simulink model "rtwdemo_ValidateLegacyCodeVrsSim"  (Simulink 7.6)
settings: Solver=FixedStepDiscrete  StartTime=0.0  StopTime=4  FixedStep=.001  RelTol=1e-3
PostLoadFcn:
  | % Load data for this model
  | rtwdemo_legacyValidationData;
undefined symbols (not defined in the file or in its folder): P_InErrMap, P_OutMap
settings Model: Creator=The MathWorks Inc.  ExtModeAutoUpdateStatusClock=off
settings OptimizationCC: InitFltsAndDblsToZero=on
settings DebuggingCC: SignalResolutionControl=TryResolveAllWithWarning  StrictBusMsg=Warning
settings GRTTargetCC: TargetFcnLib=ansi_tfl_tmw.mat

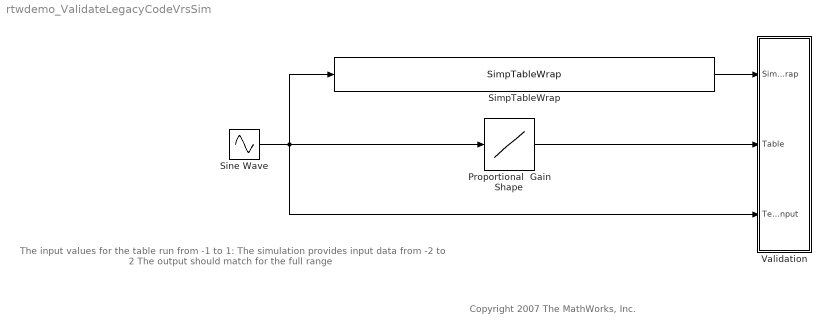
== system rtwdemo_ValidateLegacyCodeVrsSim ==
  note: The input values for the table run from -1 to 1:
      | The simulation provides input data from -2 to 2
      | The output should match for the full range
  note: Copyright 2007 The MathWorks, Inc.
  Proportional  Gain Shape : Lookup  InputValues=P_InErrMap  Table=P_OutMap  LookUpMeth=Interpolation-Use End Values
  SimpTableWrap : S-Function  FunctionName=SimpTableWrap  Parameters=SParameter1, SParameter2, SParameter3  EnableBusSupport=off  mask(Legacy Function){SFunctionSpec=double y1 = SimpleTable(double u1, double p1[], double p2[], int16 p3), SParameter1=P_InErrMap, SParameter2=P_OutMap, SParameter3=int16(length(P_OutMap)), ShowSpec=on}
      mask prompts: SParameter1 "P1:"; SParameter2 "P2:"; SParameter3 "P3:"; ShowSpec "Display function specification"
      mask help:
      | This block allows the user to call the following C function(s) in Simulink:
      |
      | StartFcn: none
      |
      | OutputFcn: double y1 = SimpleTable(double u1, double p1[], double p2[], int16 p3)
      |
      | TerminateFcn: none
      mask CallbackString:
      | ||||if strcmp(get_param(gcbh, 'ShowSpec'), 'on')
      |   set_param(gcbh, 'MaskDisplay', sprintf('fprintf(''%s'');', get_param(gcbh, 'SFunctionSpec')));
      | else
      |   set_param(gcbh, 'MaskDisplay', sprintf('fprintf(''%s'');', get_param(gcbh, 'FunctionName')));
      | end
      mask Display: fprintf('double y1 = SimpleTable(double u1, double p1[], double p2[], int16 p3)');
  Sine Wave : Sin  Amplitude=2  Frequency=pi  SampleTime=0
  Validation : Subsystem
  wires:
  SimpTableWrap/1 -> Validation/1(SimpleWrap)
  Sine Wave/1 -> SimpTableWrap/1, Proportional  Gain Shape/1, Validation/3(TestInput)
  Proportional  Gain Shape/1 -> Validation/2(Table)

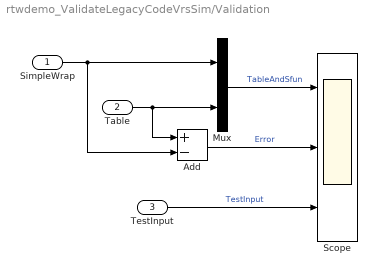
== system rtwdemo_ValidateLegacyCodeVrsSim/Validation ==
  SimpleWrap : Inport
  Table : Inport  Port=2
  TestInput : Inport  Port=3
  Add : Sum  Inputs=+-
  Mux : Mux  Inputs=2
  Scope : Scope  NumInputPorts=3
      settings: YMin=-0.1~-1~-2  YMax=1.1~1~2  SampleInput=on  SampleTime=.001
  wires:
  Mux/1 -> Scope/1  "TableAndSfun"
  SimpleWrap/1 -> Mux/1, Add/2
  Table/1 -> Mux/2, Add/1
  Add/1 -> Scope/2  "Error"
  TestInput/1 -> Scope/3  "TestInput"
